simulink model "MPC_motor_single_phase"  (R2019a)
settings: Solver=VariableStepAuto  StartTime=0.0  StopTime=inf  RelTol=1e-3
undefined symbols (not defined in the file or in its folder): L, R, Vdc
libraries: powerlib x8
settings Model: Creator=Vu Hung Dung  LastModifiedBy=Vu Hung Dung

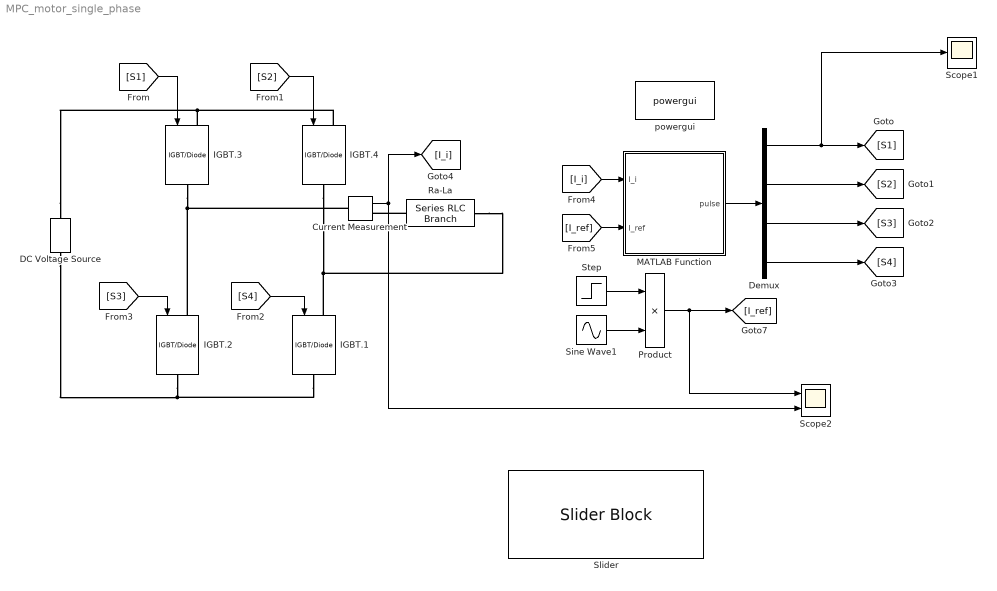
== system MPC_motor_single_phase ==
  Current Measurement : powerlib/Measurements/Current Measurement  PhasorSimulation=off  OutputType=Complex  PSBequivalent=0
      settings: SourceProductName=Simscape Electrical
  DC Voltage Source : powerlib/Electrical Sources/DC Voltage Source  Amplitude=Vdc  Measurements=Voltage
      settings: SourceProductName=Simscape Electrical
  Demux : Demux
  IGBT.{1..4} (4 alike) : powerlib/Power Electronics/IGBT//Diode  Ron=1e-3  Rs=1e5  Cs=inf  Measurements=off
      settings: SourceProductName=Simscape Electrical
  MATLAB Function : MATLAB Function  TreatAsAtomicUnit=on
  Product : Product
  Ra-La : powerlib/Elements/Series RLC Branch  LConnTagsString=__new0  RConnTagsString=__new0  BranchType=RL  Resistance=R  Inductance=L  SetiL0=off  InitialCurrent=0  Capacitance=1.0  Setx0=off  InitialVoltage=0  Measurements=None
      settings: SourceProductName=Simscape Electrical
  Scope1 : Scope
  Scope2 : Scope  NumInputPorts=2
  Sine Wave1 : Sin  Frequency=80  SampleTime=1e-4
  Slider : SliderBlock
  Step : Step  Time=0.05  Before=0.1  After=0.15  SampleTime=1e-4
  powergui : powerlib/powergui  Priority=1  SimulationMode=Discrete  SampleTime=0.0001  frequency=60  Iterations=50  frequencyindice=0  Pbase=100e6  ErrMax=1e-4  UnitsV=kV  UnitsW=MW  buscounter=0  FunctionMessages=off  echomessages=off  EnableUseOfTLC=off  CurrentSourceSwitches=off  DisableSnubberDevices=off  DisableRonSwitches=off  DisableVfSwitches=off  DisplayEquations=off  AutomaticDiscreteSolvers=off  SolverType=Tustin/Backward Euler (TBE)  Interpol=off  ExternalGateDelay=off  methode=off  Ts=100  x0status=blocks  SPID=on  SwTol=0  HookPort=off  NonlinearTolerance=0  nMaxIteration=15  ContinueOnMaxIteration=off  RestoreLinks=warning  ResistiveCurrentMeasurement=off  Frange=[0:2:500]  Ylog=off  Xlog=on  ShowGrid=off  save=off  variable=ZData  structure=0  ZoomFFT=off  StartTime=0.0  cycles=1  DisplayStyle=1  fundamental=60  FreqAxis=off  MaxFrequency=1000  frequencyindicesteady=1  RmsSteady=1  display=off
      settings: SourceProductName=Simscape Electrical
  wires:
  [S1] -> IGBT.3/1
  [S3] -> IGBT.2/1
  [S4] -> IGBT.1/1
  [S2] -> IGBT.4/1
  MATLAB Function/1(pulse) -> Demux/1
  Demux/1 -> Scope1/1, [S1]
  Demux/2 -> [S2]
  Demux/3 -> [S3]
  Demux/4 -> [S4]
  Current Measurement/1 -> Scope2/2, [I_i]
  [I_i] -> MATLAB Function/1(I_i)
  Step/1 -> Product/1
  Product/1 -> Scope2/1, [I_ref]
  Sine Wave1/1 -> Product/2
  [I_ref] -> MATLAB Function/2(I_ref)
  connections:
  DC Voltage Source/RConn1 -- IGBT.4/LConn1 -- IGBT.3/LConn1
  DC Voltage Source/LConn1 -- IGBT.1/RConn1 -- IGBT.2/RConn1
  Current Measurement/LConn1 -- IGBT.2/LConn1 -- IGBT.3/RConn1
  IGBT.1/LConn1 -- IGBT.4/RConn1 -- Ra-La/RConn1
  Ra-La/LConn1 -- Current Measurement/RConn1

== matlab function MPC_motor_single_phase/MATLAB Function ==
  data: I_i input; pulse output; I_ref input
function pulse = MPC(I_i, I_ref)
g_opt = inf;
L = 4;
R = 1000;
Vdc = 300;
Ts = 1e-4;
S1_opt = 0;
S2_opt = 0;
for S1 = 0:1
    for S2 = 0:1
        U1 = S1*Vdc;
        U2 = S2*Vdc;
        U = U1-U2;
        I_i1 = (Ts/L)*U + ((-R*Ts + L)/L)*I_i; 
        g = abs(I_i1 - I_ref);
    if (g < g_opt) 
        S1_opt = S1;
        S2_opt = S2;
        g_opt = g;
    end
    end  
end
S1 = S1_opt;
S2 = S2_opt;
pulse = [S1; S2; not(S1); not(S2)];
